simulink model "RobotX_ss_acoustics_1019_bbox"  (R2014a)
settings: Solver=FixedStepDiscrete  StartTime=0.0  StopTime=inf  FixedStep=.25  RelTol=1e-3
undefined symbols (not defined in the file): Com1, Com2, Com3, Com4, DiscIntNeverNeededParam, standard
libraries: xpcseriallib x14, dspmtrx3 x3, slrtlib x3, simulink x2, speedgoatlib x1, speedgoatlib_IO102 x1
(part 1 of 3)
settings Model: BufferReuse=off  Creator=wildcat  LastModifiedBy=wildcat
settings SolverCC: EnableConcurrentExecution=on
settings DataIOCC: SignalLoggingSaveFormat=ModelDataLogs
settings OptimizationCC: BlockReduction=off  OptimizeBlockIOStorage=off  BufferReuse=off  GlobalBufferReuse=off  ExpressionFolding=off  LocalBlockOutputs=off
settings DebuggingCC: UnderspecifiedInitializationDetection=Classic  StateNameClashWarn=warning
settings HardwareCC: ProdIntDivRoundTo=Zero  ProdEndianess=LittleEndian  ProdHWDeviceType=Generic->32-bit x86 compatible
settings RTWCC: SystemTargetFile=slrt.tlc  TemplateMakefile=slrt_default_tmf  Description=Simulink Real-Time  ProcessScript=slrt_make_rtw_hook  RTWCompilerOptimization=On
settings SimulinkRealTimeCC: GeneratePreprocessorConditionals=Disable all  EnableShiftOperators=on

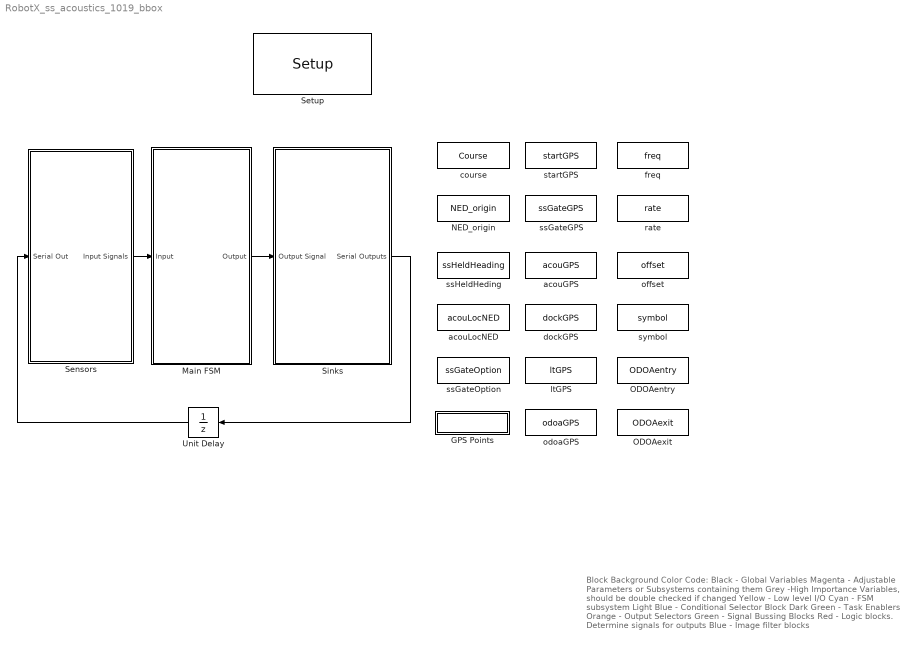
== system RobotX_ss_acoustics_1019_bbox ==
  note: Block Background Color Code:
      | Black - Global Variables
      | Magenta - Adjustable Parameters or Subsystems containing them
      | Grey -High Importance Variables, should be double checked if changed
      | Yellow - Low level I/O
      | Cyan - FSM subsystem
      | Light Blue - Conditional Selector Block
      | Dark Green - Task Enablers
      | Orange - Output Selectors
      | Green - Signal Bussing Blocks
      | Red - Logic blocks. Determine signals for outputs
      | Blue - Image filter blocks
  GPS Points : Subsystem
  Main FSM : Subsystem
  NED_origin : DataStoreMemory  DataStoreName=NED_origin  ReadBeforeWriteMsg=warning  WriteAfterWriteMsg=warning  WriteAfterReadMsg=warning  InitialValue="[1.2879,  103.8584]"  VectorParams1D=off
  ODOAentry : DataStoreMemory  DataStoreName=ODOAentry  ReadBeforeWriteMsg=warning  WriteAfterWriteMsg=warning  WriteAfterReadMsg=warning  VectorParams1D=off
  ODOAexit : DataStoreMemory  DataStoreName=ODOAexit  ReadBeforeWriteMsg=warning  WriteAfterWriteMsg=warning  WriteAfterReadMsg=warning  VectorParams1D=off
  Sensors : Subsystem
  Setup : speedgoatlib_IO102/Setup  group=Digital output setup  id=1  range=+-5V  cal=off  pciSlot=-1  adChannelMode=Multiple-channel (enter number of channels below)  adChannel=16  adCoupling=Differential  daChannel=[1,2,3,4]  daReset=[1]  daInitValue=[0]  diChannel=[1,2,3,4,5,6,7,8]  doChannel=[1,2,3,4,5,6,7,8]  doReset=[1]  doInitValue=[0]
  Sinks : Subsystem
  Unit Delay : UnitDelay  SampleTime=-1
  acouGPS : DataStoreMemory  DataStoreName=acouGPS  ReadBeforeWriteMsg=warning  WriteAfterWriteMsg=warning  WriteAfterReadMsg=warning  InitialValue=zeros(4,2)  VectorParams1D=off
  acouLocNED : DataStoreMemory  DataStoreName=acouLocNED  ReadBeforeWriteMsg=warning  WriteAfterWriteMsg=warning  WriteAfterReadMsg=warning  InitialValue=[45, -180; 60, -160; 75, -175]  VectorParams1D=off
  course : DataStoreMemory  DataStoreName=Course  ReadBeforeWriteMsg=warning  WriteAfterWriteMsg=warning  WriteAfterReadMsg=warning  InitialValue=uint8('A')  VectorParams1D=off
  dockGPS : DataStoreMemory  DataStoreName=dockGPS  ReadBeforeWriteMsg=warning  WriteAfterWriteMsg=warning  WriteAfterReadMsg=warning  InitialValue=zeros(4,2)  VectorParams1D=off
  freq : DataStoreMemory  DataStoreName=freq  ReadBeforeWriteMsg=warning  WriteAfterWriteMsg=warning  WriteAfterReadMsg=warning  VectorParams1D=off
  ltGPS : DataStoreMemory  DataStoreName=ltGPS  ReadBeforeWriteMsg=warning  WriteAfterWriteMsg=warning  WriteAfterReadMsg=warning  InitialValue=zeros(4,2)  VectorParams1D=off
  odoaGPS : DataStoreMemory  DataStoreName=odoaGPS  ReadBeforeWriteMsg=warning  WriteAfterWriteMsg=warning  WriteAfterReadMsg=warning  InitialValue=zeros(4,2)  VectorParams1D=off
  offset : DataStoreMemory  DataStoreName=offset  ReadBeforeWriteMsg=warning  WriteAfterWriteMsg=warning  WriteAfterReadMsg=warning  VectorParams1D=off
  rate : DataStoreMemory  DataStoreName=rate  ReadBeforeWriteMsg=warning  WriteAfterWriteMsg=warning  WriteAfterReadMsg=warning  VectorParams1D=off
  ssGateGPS : DataStoreMemory  DataStoreName=ssGateGPS  ReadBeforeWriteMsg=warning  WriteAfterWriteMsg=warning  WriteAfterReadMsg=warning  InitialValue=zeros(4,2)  VectorParams1D=off
  ssGateOption : DataStoreMemory  DataStoreName=ssGateOption  ReadBeforeWriteMsg=warning  WriteAfterWriteMsg=warning  WriteAfterReadMsg=warning  VectorParams1D=off
  ssHeldHeding : DataStoreMemory  DataStoreName=ssHeldHeading  ReadBeforeWriteMsg=warning  WriteAfterWriteMsg=warning  WriteAfterReadMsg=warning
  startGPS : DataStoreMemory  DataStoreName=startGPS  ReadBeforeWriteMsg=warning  WriteAfterWriteMsg=warning  WriteAfterReadMsg=warning  InitialValue=zeros(1,2)  VectorParams1D=off
  symbol : DataStoreMemory  DataStoreName=symbol  ReadBeforeWriteMsg=warning  WriteAfterWriteMsg=warning  WriteAfterReadMsg=warning  VectorParams1D=off
  wires:
  Main FSM/1(Output) -> Sinks/1(Output Signal)
  Sensors/1(Input Signals) -> Main FSM/1(Input)
  Sinks/1(Serial Outputs) -> Unit Delay/1
  Unit Delay/1 -> Sensors/1(Serial Out)

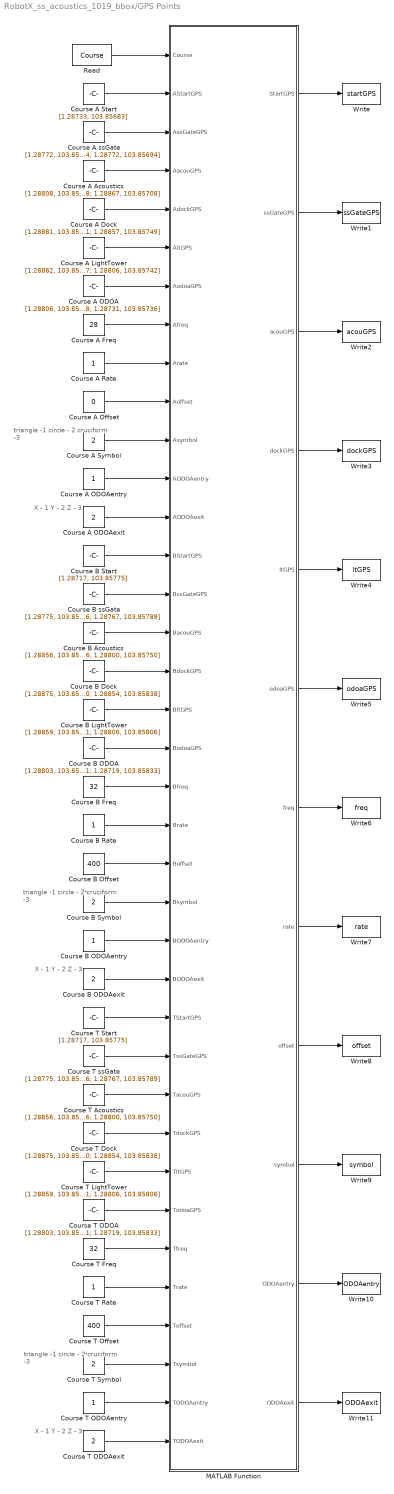
== system RobotX_ss_acoustics_1019_bbox/GPS Points ==
  note: X - 1
      | Y - 2
      | Z - 3
  note: triangle -1
      | circle - 2
      | cruciform -3
  note: X - 1
      | Y - 2
      | Z - 3
  note: triangle -1
      | circle - 2
      | cruciform -3
  note: X - 1
      | Y - 2
      | Z - 3
  note: triangle -1
      | circle - 2
      | cruciform -3
  Course A Acoustics : Constant  Value=[1.28808, 103.85714; 1.28869, 103.85669; 1.28817, 103.85658; 1.28867, 103.85708]  VectorParams1D=off
  Course A Dock : Constant  Value=[1.28881, 103.85717; 1.28875, 103.85753; 1.28862, 103.85721; 1.28857, 103.85749]  VectorParams1D=off
  Course A Freq : Constant  Value=28  VectorParams1D=off
  Course A LightTower : Constant  Value=[1.28862, 103.85721; 1.28857, 103.85749; 1.28806, 103.85717; 1.28806, 103.85742]  VectorParams1D=off
  Course A ODOA : Constant  Value=[1.28806, 103.85717; 1.28806, 103.85742; 1.28733, 103.85708; 1.28731, 103.85736]  VectorParams1D=off
  Course A ODOAentry : Constant  VectorParams1D=off
  Course A ODOAexit : Constant  Value=2  VectorParams1D=off
  Course A Offset : Constant  Value=0  VectorParams1D=off
  Course A Rate : Constant  VectorParams1D=off
  Course A Start : Constant  Value=[1.28733, 103.85683]  VectorParams1D=off
  Course A Symbol : Constant  Value=2  VectorParams1D=off
  Course A ssGate : Constant  Value=[1.28772, 103.85675; 1.28739, 103.85675; 1.28739, 103.85694; 1.28772, 103.85694]  VectorParams1D=off
  Course B Acoustics : Constant  Value=[1.28856, 103.85761; 1.28867, 103.85794; 1.28800, 103.85786; 1.28800, 103.85750]  VectorParams1D=off
  Course B Dock : Constant  Value=[1.28875, 103.85811; 1.28869, 103.85844; 1.28859, 103.85810; 1.28854, 103.85838]  VectorParams1D=off
  Course B Freq : Constant  Value=32  VectorParams1D=off
  Course B LightTower : Constant  Value=[1.28859, 103.85810; 1.28854, 103.85838; 1.28803, 103.85831; 1.28806, 103.85806]  VectorParams1D=off
  Course B ODOA : Constant  Value=[1.28803, 103.85831; 1.28806, 103.85806; 1.28722, 103.85811; 1.28719, 103.85833]  VectorParams1D=off
  Course B ODOAentry : Constant  VectorParams1D=off
  Course B ODOAexit : Constant  Value=2  VectorParams1D=off
  Course B Offset : Constant  Value=400  VectorParams1D=off
  Course B Rate : Constant  VectorParams1D=off
  Course B Start : Constant  Value=[1.28717, 103.85775]  VectorParams1D=off
  Course B Symbol : Constant  Value=2  VectorParams1D=off
  Course B ssGate : Constant  Value=[1.28775, 103.85761; 1.28725, 103.85764; 1.28719, 103.85786; 1.28767, 103.85789]  VectorParams1D=off
  Course T Acoustics : Constant  Value=[1.28856, 103.85761; 1.28867, 103.85794; 1.28800, 103.85786; 1.28800, 103.85750]  VectorParams1D=off
  Course T Dock : Constant  Value=[1.28875, 103.85811; 1.28869, 103.85844; 1.28859, 103.85810; 1.28854, 103.85838]  VectorParams1D=off
  Course T Freq : Constant  Value=32  VectorParams1D=off
  Course T LightTower : Constant  Value=[1.28859, 103.85810; 1.28854, 103.85838; 1.28803, 103.85831; 1.28806, 103.85806]  VectorParams1D=off
  Course T ODOA : Constant  Value=[1.28803, 103.85831; 1.28806, 103.85806; 1.28722, 103.85811; 1.28719, 103.85833]  VectorParams1D=off
  Course T ODOAentry : Constant  VectorParams1D=off
  Course T ODOAexit : Constant  Value=2  VectorParams1D=off
  Course T Offset : Constant  Value=400  VectorParams1D=off
  Course T Rate : Constant  VectorParams1D=off
  Course T Start : Constant  Value=[1.28717, 103.85775]  VectorParams1D=off
  Course T Symbol : Constant  Value=2  VectorParams1D=off
  Course T ssGate : Constant  Value=[1.28775, 103.85761; 1.28725, 103.85764; 1.28719, 103.85786; 1.28767, 103.85789]  VectorParams1D=off
  MATLAB Function : MATLAB Function  TreatAsAtomicUnit=on
  Read : DataStoreRead  DataStoreName=Course
  Write : DataStoreWrite  DataStoreName=startGPS
  Write1 : DataStoreWrite  DataStoreName=ssGateGPS
  Write10 : DataStoreWrite  DataStoreName=ODOAentry
  Write11 : DataStoreWrite  DataStoreName=ODOAexit
  Write2 : DataStoreWrite  DataStoreName=acouGPS
  Write3 : DataStoreWrite  DataStoreName=dockGPS
  Write4 : DataStoreWrite  DataStoreName=ltGPS
  Write5 : DataStoreWrite  DataStoreName=odoaGPS
  Write6 : DataStoreWrite  DataStoreName=freq
  Write7 : DataStoreWrite  DataStoreName=rate
  Write8 : DataStoreWrite  DataStoreName=offset
  Write9 : DataStoreWrite  DataStoreName=symbol
  wires:
  Course T LightTower/1 -> MATLAB Function/30(TltGPS)
  Course T Rate/1 -> MATLAB Function/33(Trate)
  Course T Symbol/1 -> MATLAB Function/35(Tsymbol)
  Course T ODOA/1 -> MATLAB Function/31(TodoaGPS)
  Course T Freq/1 -> MATLAB Function/32(Tfreq)
  Course T Offset/1 -> MATLAB Function/34(Toffset)
  Course T ODOAexit/1 -> MATLAB Function/37(TODOAexit)
  Course T Dock/1 -> MATLAB Function/29(TdockGPS)
  Course T Acoustics/1 -> MATLAB Function/28(TacouGPS)
  Course T ODOAentry/1 -> MATLAB Function/36(TODOAentry)
  Course T Start/1 -> MATLAB Function/26(TStartGPS)
  Course T ssGate/1 -> MATLAB Function/27(TssGateGPS)
  Course B ODOAexit/1 -> MATLAB Function/25(BODOAexit)
  Course B Dock/1 -> MATLAB Function/17(BdockGPS)
  Course B Rate/1 -> MATLAB Function/21(Brate)
  Course B LightTower/1 -> MATLAB Function/18(BltGPS)
  Course B Freq/1 -> MATLAB Function/20(Bfreq)
  Course B Symbol/1 -> MATLAB Function/23(Bsymbol)
  Course B ODOA/1 -> MATLAB Function/19(BodoaGPS)
  Course B ODOAentry/1 -> MATLAB Function/24(BODOAentry)
  Course B Acoustics/1 -> MATLAB Function/16(BacouGPS)
  Course B Offset/1 -> MATLAB Function/22(Boffset)
  Course B Start/1 -> MATLAB Function/14(BStartGPS)
  Course B ssGate/1 -> MATLAB Function/15(BssGateGPS)
  Course A ODOAentry/1 -> MATLAB Function/12(AODOAentry)
  Course A Acoustics/1 -> MATLAB Function/4(AacouGPS)
  Course A Offset/1 -> MATLAB Function/10(Aoffset)
  Course A Dock/1 -> MATLAB Function/5(AdockGPS)
  Course A Freq/1 -> MATLAB Function/8(Afreq)
  Course A Rate/1 -> MATLAB Function/9(Arate)
  Course A LightTower/1 -> MATLAB Function/6(AltGPS)
  Course A ODOAexit/1 -> MATLAB Function/13(AODOAexit)
  Course A ODOA/1 -> MATLAB Function/7(AodoaGPS)
  Course A Symbol/1 -> MATLAB Function/11(Asymbol)
  Course A ssGate/1 -> MATLAB Function/3(AssGateGPS)
  Course A Start/1 -> MATLAB Function/2(AStartGPS)
  Read/1 -> MATLAB Function/1(Course)
  MATLAB Function/1(StartGPS) -> Write/1
  MATLAB Function/2(ssGateGPS) -> Write1/1
  MATLAB Function/3(acouGPS) -> Write2/1
  MATLAB Function/4(dockGPS) -> Write3/1
  MATLAB Function/5(ltGPS) -> Write4/1
  MATLAB Function/6(odoaGPS) -> Write5/1
  MATLAB Function/7(freq) -> Write6/1
  MATLAB Function/8(rate) -> Write7/1
  MATLAB Function/9(offset) -> Write8/1
  MATLAB Function/10(symbol) -> Write9/1
  MATLAB Function/11(ODOAentry) -> Write10/1
  MATLAB Function/12(ODOAexit) -> Write11/1

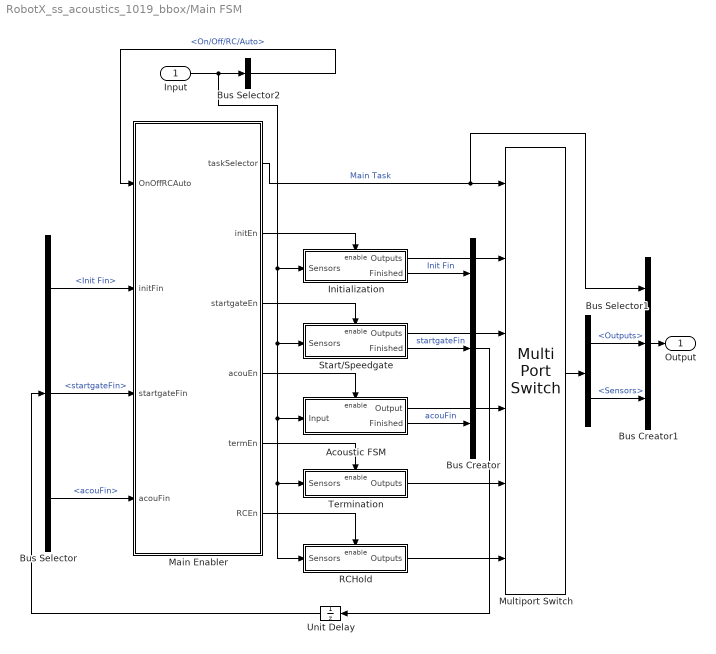
== system RobotX_ss_acoustics_1019_bbox/Main FSM ==
  Input : Inport
  Acoustic FSM : Subsystem
  Bus Creator : BusCreator  Inputs=3
  Bus Creator1 : BusCreator  Inputs=3
  Bus Selector : BusSelector  OutputSignals=Init Fin,startgateFin,acouFin
  Bus Selector1 : BusSelector  OutputSignals=Outputs,Sensors
  Bus Selector2 : BusSelector  OutputSignals=Navigation Message.On/Off/RC/Auto
  Initialization : Subsystem
  Main Enabler : MATLAB Function  TreatAsAtomicUnit=on
  Multiport Switch : MultiPortSwitch  Inputs=5
  RCHold : Subsystem
  Start/Speedgate : Subsystem  TreatAsAtomicUnit=on
  Termination : Subsystem
  Unit Delay : UnitDelay  SampleTime=-1
  Output : Outport
  wires:
  Input/1 -> Initialization/1(Sensors), Acoustic FSM/1(Input), Termination/1(Sensors), RCHold/1(Sensors), Start/Speedgate/1(Sensors), Bus Selector2/1
  Bus Selector2/1 -> Main Enabler/1(OnOffRCAuto)  "<On/Off/RC/Auto>"
  RCHold/1(Outputs) -> Multiport Switch/6
  Main Enabler/2(initEn) -> Initialization/Enable
  Main Enabler/3(startgateEn) -> Start/Speedgate/Enable
  Main Enabler/6(RCEn) -> RCHold/Enable
  Main Enabler/1(taskSelector) -> Bus Creator1/1, Multiport Switch/1  "Main Task"
  Multiport Switch/1 -> Bus Selector1/1
  Unit Delay/1 -> Bus Selector/1
  Termination/1(Outputs) -> Multiport Switch/5
  Main Enabler/5(termEn) -> Termination/Enable
  Bus Creator/1 -> Unit Delay/1
  Bus Selector/1 -> Main Enabler/2(initFin)  "<Init Fin>"
  Bus Selector/2 -> Main Enabler/3(startgateFin)  "<startgateFin>"
  Acoustic FSM/1(Output) -> Multiport Switch/4
  Main Enabler/4(acouEn) -> Acoustic FSM/Enable
  Start/Speedgate/1(Outputs) -> Multiport Switch/3
  Initialization/1(Outputs) -> Multiport Switch/2
  Initialization/2(Finished) -> Bus Creator/1  "Init Fin"
  Start/Speedgate/2(Finished) -> Bus Creator/2  "startgateFin"
  Acoustic FSM/2(Finished) -> Bus Creator/3  "acouFin"
  Bus Selector/3 -> Main Enabler/4(acouFin)  "<acouFin>"
  Bus Creator1/1 -> Output/1
  Bus Selector1/1 -> Bus Creator1/2  "<Outputs>"
  Bus Selector1/2 -> Bus Creator1/3  "<Sensors>"

== system RobotX_ss_acoustics_1019_bbox/Sensors ==
  Serial Out : Inport
  Serial In : Subsystem
  Input Signals : Outport
  wires:
  Serial In/1(Serial In) -> Input Signals/1  "Sensors"
  Serial Out/1 -> Serial In/1(Serial Out)

== system RobotX_ss_acoustics_1019_bbox/Sinks ==
  Output Signal : Inport
  Serial Outputs : Outport
  wires:
  Output Signal/1 -> Serial Outputs/1

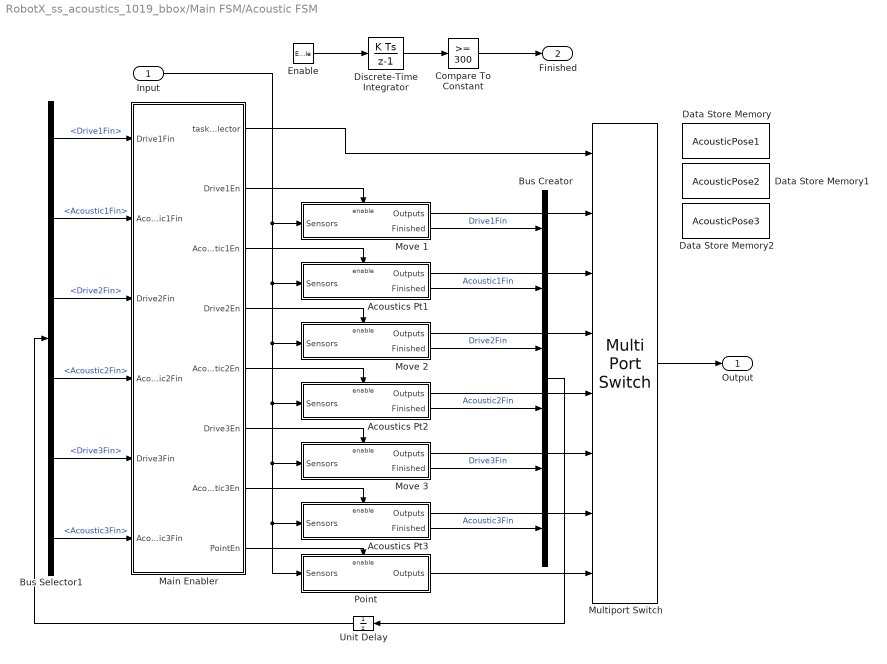
== system RobotX_ss_acoustics_1019_bbox/Main FSM/Acoustic FSM ==
  Input : Inport
  Enable : EnablePort  ShowOutputPort=on
  Acoustics Pt1 : Subsystem  TreatAsAtomicUnit=on
  Acoustics Pt2 : Subsystem  TreatAsAtomicUnit=on
  Acoustics Pt3 : Subsystem  TreatAsAtomicUnit=on
  Bus Creator : BusCreator  Inputs=6
  Bus Selector1 : BusSelector  OutputSignals=Drive1Fin,Acoustic1Fin,Drive2Fin,Acoustic2Fin,Drive3Fin,Acoustic3Fin
  Compare To Constant : simulink/Logic and Bit Operations/Compare To Constant  relop=>=  const=300  OutDataTypeStr=boolean
  Data Store Memory : DataStoreMemory  DataStoreName=AcousticPose1  ReadBeforeWriteMsg=warning  WriteAfterWriteMsg=warning  WriteAfterReadMsg=warning  InitialValue=[0 0 0]
  Data Store Memory1 : DataStoreMemory  DataStoreName=AcousticPose2  ReadBeforeWriteMsg=warning  WriteAfterWriteMsg=warning  WriteAfterReadMsg=warning  InitialValue=[0 0 0]
  Data Store Memory2 : DataStoreMemory  DataStoreName=AcousticPose3  ReadBeforeWriteMsg=warning  WriteAfterWriteMsg=warning  WriteAfterReadMsg=warning  InitialValue=[0 0 0]
  Discrete-Time Integrator : DiscreteIntegrator  SampleTime=-1  ICPrevOutput=DiscIntNeverNeededParam  ICPrevScaledInput=DiscIntNeverNeededParam
  Main Enabler : MATLAB Function  TreatAsAtomicUnit=on
  Move 1 : Subsystem
  Move 2 : Subsystem
  Move 3 : Subsystem
  Multiport Switch : MultiPortSwitch  Inputs=7
  Point : Subsystem  TreatAsAtomicUnit=on
  Unit Delay : UnitDelay  SampleTime=-1
  Output : Outport
  Finished : Outport  Port=2
  wires:
  Input/1 -> Move 1/1(Sensors), Acoustics Pt1/1(Sensors), Move 2/1(Sensors), Acoustics Pt2/1(Sensors), Move 3/1(Sensors), Acoustics Pt3/1(Sensors), Point/1(Sensors)
  Multiport Switch/1 -> Output/1
  Unit Delay/1 -> Bus Selector1/1
  Move 1/1(Outputs) -> Multiport Switch/2
  Move 1/2(Finished) -> Bus Creator/1  "Drive1Fin"
  Acoustics Pt1/2(Finished) -> Bus Creator/2  "Acoustic1Fin"
  Move 2/2(Finished) -> Bus Creator/3  "Drive2Fin"
  Acoustics Pt2/2(Finished) -> Bus Creator/4  "Acoustic2Fin"
  Move 3/2(Finished) -> Bus Creator/5  "Drive3Fin"
  Acoustics Pt3/2(Finished) -> Bus Creator/6  "Acoustic3Fin"
  Bus Creator/1 -> Unit Delay/1
  Main Enabler/2(Drive1En) -> Move 1/Enable
  Main Enabler/3(Acoustic1En) -> Acoustics Pt1/Enable
  Main Enabler/4(Drive2En) -> Move 2/Enable
  Main Enabler/5(Acoustic2En) -> Acoustics Pt2/Enable
  Main Enabler/6(Drive3En) -> Move 3/Enable
  Main Enabler/7(Acoustic3En) -> Acoustics Pt3/Enable
  Main Enabler/8(PointEn) -> Point/Enable
  Bus Selector1/6 -> Main Enabler/6(Acoustic3Fin)  "<Acoustic3Fin>"
  Bus Selector1/4 -> Main Enabler/4(Acoustic2Fin)  "<Acoustic2Fin>"
  Bus Selector1/2 -> Main Enabler/2(Acoustic1Fin)  "<Acoustic1Fin>"
  Bus Selector1/5 -> Main Enabler/5(Drive3Fin)  "<Drive3Fin>"
  Bus Selector1/3 -> Main Enabler/3(Drive2Fin)  "<Drive2Fin>"
  Bus Selector1/1 -> Main Enabler/1(Drive1Fin)  "<Drive1Fin>"
  Acoustics Pt1/1(Outputs) -> Multiport Switch/3
  Move 2/1(Outputs) -> Multiport Switch/4
  Acoustics Pt2/1(Outputs) -> Multiport Switch/5
  Move 3/1(Outputs) -> Multiport Switch/6
  Acoustics Pt3/1(Outputs) -> Multiport Switch/7
  Point/1(Outputs) -> Multiport Switch/8
  Main Enabler/1(taskSelector) -> Multiport Switch/1
  Enable/1 -> Discrete-Time Integrator/1
  Discrete-Time Integrator/1 -> Compare To Constant/1
  Compare To Constant/1 -> Finished/1

== system RobotX_ss_acoustics_1019_bbox/Main FSM/Initialization ==
  Sensors : Inport
  Enable : EnablePort  ShowOutputPort=on
  Compare To Constant : simulink/Logic and Bit Operations/Compare To Constant  relop=>=  const=50  OutDataTypeStr=boolean
  Data Type Conversion : DataTypeConversion  OutDataTypeStr=double
  Discrete-Time Integrator : DiscreteIntegrator  SampleTime=-1  ICPrevOutput=DiscIntNeverNeededParam  ICPrevScaledInput=DiscIntNeverNeededParam
  Output Heirarchy : Subsystem
  Outputs : Outport
  Finished : Outport  Port=2
  wires:
  Sensors/1 -> Output Heirarchy/1(Sensors)
  Output Heirarchy/1(Outputs) -> Outputs/1
  Compare To Constant/1 -> Data Type Conversion/1
  Enable/1 -> Discrete-Time Integrator/1
  Discrete-Time Integrator/1 -> Compare To Constant/1
  Data Type Conversion/1 -> Finished/1

== system RobotX_ss_acoustics_1019_bbox/Main FSM/RCHold ==
  Sensors : Inport
  Enable : EnablePort
  Direct Control : Subsystem
  Outputs : Outport
  wires:
  Direct Control/1(Outputs) -> Outputs/1
  Sensors/1 -> Direct Control/1(Sensors)

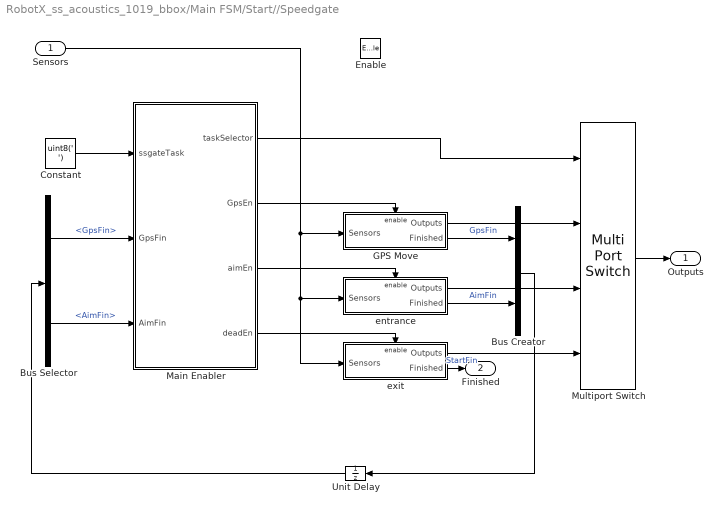
== system RobotX_ss_acoustics_1019_bbox/Main FSM/Start//Speedgate ==
  Sensors : Inport
  Enable : EnablePort
  Bus Creator : BusCreator  Inputs=2
  Bus Selector : BusSelector  OutputSignals=GpsFin,AimFin
  Constant : Constant  Value=uint8(' ')  VectorParams1D=off
  GPS Move : Subsystem
  Main Enabler : MATLAB Function  TreatAsAtomicUnit=on
  Multiport Switch : MultiPortSwitch
  Unit Delay : UnitDelay  SampleTime=-1
  entrance : Subsystem
  exit : Subsystem
  Outputs : Outport
  Finished : Outport  Port=2  InitialOutput=0
  wires:
  Main Enabler/1(taskSelector) -> Multiport Switch/1
  Constant/1 -> Main Enabler/1(ssgateTask)
  Bus Selector/1 -> Main Enabler/2(GpsFin)  "<GpsFin>"
  Unit Delay/1 -> Bus Selector/1
  Main Enabler/2(GpsEn) -> GPS Move/Enable
  Main Enabler/4(deadEn) -> exit/Enable
  Bus Creator/1 -> Unit Delay/1
  Sensors/1 -> exit/1(Sensors), entrance/1(Sensors), GPS Move/1(Sensors)
  Multiport Switch/1 -> Outputs/1
  Main Enabler/3(aimEn) -> entrance/Enable
  exit/1(Outputs) -> Multiport Switch/4
  entrance/1(Outputs) -> Multiport Switch/3
  GPS Move/1(Outputs) -> Multiport Switch/2
  GPS Move/2(Finished) -> Bus Creator/1  "GpsFin"
  entrance/2(Finished) -> Bus Creator/2  "AimFin"
  Bus Selector/2 -> Main Enabler/3(AimFin)  "<AimFin>"
  exit/2(Finished) -> Finished/1  "StartFin"

== system RobotX_ss_acoustics_1019_bbox/Main FSM/Termination ==
  Sensors : Inport
  Enable : EnablePort
  Bus Selector : BusSelector  OutputSignals=Navigation Message.Pose.X,Navigation Message.Pose.Y,Navigation Message.Pose.Psi,Navigation Message.Velocity.u
  CalcTimes : MATLAB Function  TreatAsAtomicUnit=on
  Data Store Read : DataStoreRead  DataStoreName=startGPS
  Data Store Read1 : DataStoreRead  DataStoreName=NED_origin
  GPSMove : MATLAB Function  TreatAsAtomicUnit=on
  LLA to NED : MATLAB Function  TreatAsAtomicUnit=on
  Output Reassign : Subsystem
  Outputs : Outport
  wires:
  GPSMove/2(pts) -> CalcTimes/1(pts)
  Sensors/1 -> Output Reassign/3(Sensors), Bus Selector/1
  Bus Selector/1 -> GPSMove/2(X)  "<X>"
  Bus Selector/2 -> GPSMove/3(Y)  "<Y>"
  Bus Selector/3 -> GPSMove/4(Psi)  "<Psi>"
  Bus Selector/4 -> CalcTimes/2(u)  "<u>"
  Output Reassign/1(Outputs) -> Outputs/1
  CalcTimes/1(Data) -> Output Reassign/2(Data)
  GPSMove/1(valid) -> Output Reassign/1(Vaild)
  LLA to NED/1(GoalNED) -> GPSMove/1(GoalNED)
  Data Store Read/1 -> LLA to NED/1(GoalLLA)
  Data Store Read1/1 -> LLA to NED/2(NED_origin)

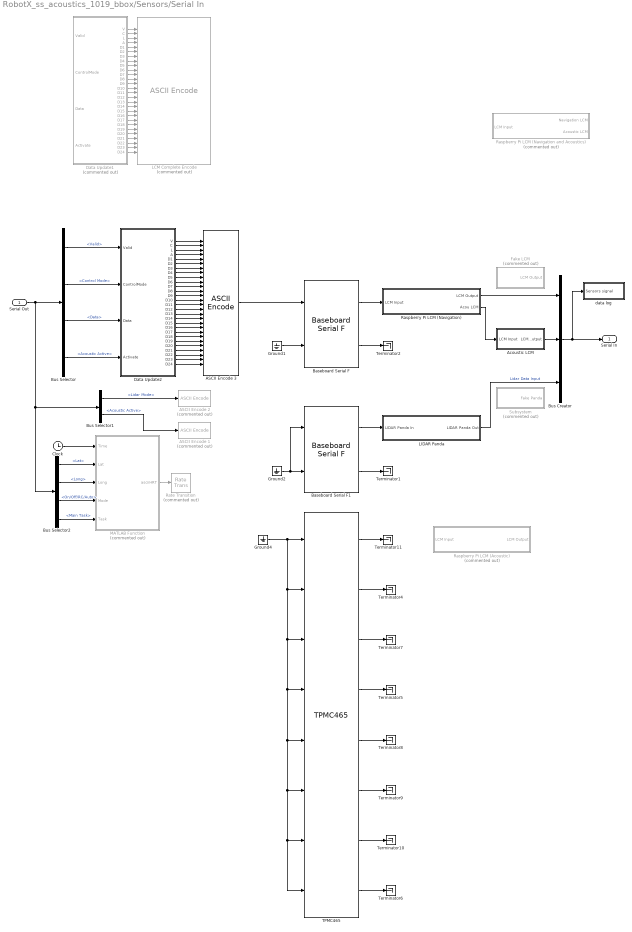
== system RobotX_ss_acoustics_1019_bbox/Sensors/Serial In ==
  Serial Out : Inport
  " Raspberry Pi LCM (Acoustic)" : Subsystem  Commented=on
  " Raspberry Pi LCM (Navigation and Acoustics)" : Subsystem  Commented=on
  " Raspberry Pi LCM (Navigation)" : Subsystem
  ASCII Encode 1 : xpcseriallib/ASCII Encode   Commented=on  format="{\"Activate\":%d} \\r\\n"  nvars=1  maxlength=20  vartypes={ 'double' }
  ASCII Encode 2 : xpcseriallib/ASCII Encode   Commented=on  format=SGTask:%d \r\n  nvars=1  maxlength=128  vartypes={ 'double' }
  ASCII Encode 3 : xpcseriallib/ASCII Encode   format="{\"Valid\":%d, \"Mode\":%d, \"Length\":%d, \"Activate\":%d, \"Waypoints\":[%f, %f, %f, %f, %f, %f, %f, %f, %f, %f, %f, %f, %f, %f, %f, %f, %f, %f, %f, %f, %f, %f, %f, %f]} \\r\\n"  nvars=28  maxlength=1000  vartypes={ 'double' }
  Acoustic LCM : Subsystem
  Baseboard Serial F : xpcseriallib/Mainboard/Baseboard Serial F  group=Basic Setup  port=1  irqnum=4  saddr1=0x3f8  saddr2=0x3e8  config=Com1/Com3  baud1=115200  parity1=Even  ndata1=7  nstop1=1  fifomode1=64 deep  rlevel1=quarter full  automode1=on  xmtfifosize1=1024  xmtdatatype1=8 bit uint null terminated  rcvfifosize1=1024  baud2=115200  parity2=Even  ndata2=7  nstop2=1  fifomode2=64 deep  rlevel2=1  automode2=on  xmtfifosize2=1024  xmtdatatype2=8 bit uint null terminated  rcvfifosize2=1024
  Baseboard Serial F1 : xpcseriallib/Mainboard/Baseboard Serial F  group=Basic Setup  port=2  irqnum=4  saddr1=0x3f8  saddr2=0x3e8  config=Com2/Com4  baud1=115200  parity1=Even  ndata1=7  nstop1=1  fifomode1=64 deep  rlevel1=quarter full  automode1=on  xmtfifosize1=1024  xmtdatatype1=8 bit uint null terminated  rcvfifosize1=1024  baud2=115200  parity2=Even  ndata2=7  nstop2=1  fifomode2=64 deep  rlevel2=quarter full  automode2=on  xmtfifosize2=1024  xmtdatatype2=8 bit uint null terminated  rcvfifosize2=1024
  Bus Creator : BusCreator  Inputs=3
  Bus Selector : BusSelector  OutputSignals=Outputs.Navigation Outputs.Valid,Outputs.Navigation Outputs.Control Mode,Outputs.Navigation Outputs.Data,Outputs.Acoustic Active
  Bus Selector1 : BusSelector  OutputSignals=Outputs.Lidar Mode,Outputs.Acoustic Active
  Bus Selector2 : BusSelector  OutputSignals=Sensors.Navigation Message.GPS (LLA).Lat,Sensors.Navigation Message.GPS (LLA).Long,Sensors.Navigation Message.On/Off/RC/Auto,Main Task
  Clock : Clock
  Data Update1 : MATLAB Function  Commented=on  TreatAsAtomicUnit=on
  Data Update2 : MATLAB Function  TreatAsAtomicUnit=on
  Fake LCM : Subsystem  Commented=on
  Ground1 : Ground
  Ground2 : Ground
  Ground4 : Ground
  LCM Complete Encode : xpcseriallib/ASCII Encode   Commented=on  format="{\"Valid\":%d, \"Mode\":%d, \"Length\":%d, \"Activate\":%d, \"Waypoints\":[%f, %f, %f, %f, %f, %f, %f, %f, %f, %f, %f, %f, %f, %f, %f, %f, %f, %f, %f, %f, %f, %f, %f, %f]} \\r\\n"  nvars=28  maxlength=1000  vartypes={ 'double' }
  LIDAR Panda : Subsystem
  MATLAB Function : MATLAB Function  Commented=on  TreatAsAtomicUnit=on
  Rate Transition : RateTransition  Commented=on  Deterministic=off  OutPortSampleTime=1
  Subsystem : Subsystem  Commented=on
  TPMC465 : speedgoatlib/IO504/TPMC465  group=Basic Setup  port=2  irqnum=9  slot=-1  transceiver1=RS232 (max 921.6kb/s)  standard1=on  baud1=115200  bauddivisor1=1  sampling1=16x (standard)  prescale1=off  parity1=Even  ndata1=7  nstop1=1  rlevel1=half full (32)  hwmode1=none  swmode1=none  xonchar1=17  xoffchar1=19  rs485auto1=off  rs485delay1=0  xmtfifosize1=1024  xmtdatatype1=8 bit uint null terminated  rcvfifosize1=1024  transceiver2=RS232 (max 921.6kb/s)  standard2=on  baud2=115200  bauddivisor2=1  sampling2=16x (standard)  prescale2=off  parity2=Even  ndata2=7  nstop2=1  rlevel2=1  hwmode2=none  swmode2=none  xonchar2=17  xoffchar2=19  rs485auto2=off  rs485delay2=0  xmtfifosize2=1024  xmtdatatype2=8 bit uint null terminated  rcvfifosize2=1024  transceiver3=RS232 (max 921.6kb/s)  standard3=on  baud3=115200  bauddivisor3=1  sampling3=16x (standard)  prescale3=off  parity3=None  ndata3=8  nstop3=1  rlevel3=half full (32)  hwmode3=none  swmode3=none  xonchar3=17  xoffchar3=19  rs485auto3=off  rs485delay3=0  xmtfifosize3=1024  xmtdatatype3=8 bit uint null terminated  rcvfifosize3=1024  transceiver4=RS232 (max 921.6kb/s)  standard4=on  baud4=115200  bauddivisor4=1  sampling4=16x (standard)  prescale4=off  parity4=None  ndata4=8  nstop4=1  rlevel4=half full (32)  hwmode4=none  swmode4=none  xonchar4=17  xoffchar4=19  rs485auto4=off  rs485delay4=0  xmtfifosize4=1024  xmtdatatype4=8 bit uint null terminated  rcvfifosize4=1024  transceiver5=RS232 (max 921.6kb/s)  standard5=on  baud5=115200  bauddivisor5=1  sampling5=16x (standard)  prescale5=off  parity5=None  ndata5=8  nstop5=1  rlevel5=1  hwmode5=none  swmode5=none  xonchar5=17  xoffchar5=19  rs485auto5=off  rs485delay5=0  xmtfifosize5=1024  xmtdatatype5=8 bit uint null terminated  rcvfifosize5=1024  transceiver6=RS232 (max 921.6kb/s)  standard6=on  baud6=115200  bauddivisor6=1  sampling6=16x (standard)  prescale6=off  parity6=None  ndata6=8  nstop6=1  rlevel6=1  hwmode6=none  swmode6=none  xonchar6=17  xoffchar6=19  rs485auto6=off  rs485delay6=0  xmtfifosize6=1024  xmtdatatype6=8 bit uint null terminated  rcvfifosize6=1024  transceiver7=RS232 (max 921.6kb/s)  standard7=on  baud7=115200  bauddivisor7=1  sampling7=16x (standard)  prescale7=off  parity7=None  ndata7=8  nstop7=1  rlevel7=1  hwmode7=none  swmode7=none  xonchar7=17  xoffchar7=19  rs485auto7=off  rs485delay7=0  xmtfifosize7=1024  xmtdatatype7=8 bit uint null terminated  rcvfifosize7=1024  transceiver8=RS232 (max 921.6kb/s)  standard8=on  baud8=115200  bauddivisor8=1  sampling8=16x (standard)  prescale8=off  parity8=None  ndata8=8  nstop8=1  rlevel8=1  hwmode8=none  swmode8=none  xonchar8=17  xoffchar8=19  rs485auto8=off  rs485delay8=0  xmtfifosize8=1024  xmtdatatype8=8 bit uint null terminated  rcvfifosize8=1024
  Terminator{1..2,4..11} (10 alike) : Terminator
  data log : Subsystem
  Serial In : Outport
  wires:
  Baseboard Serial F1/1 -> LIDAR Panda/1(LIDAR Panda In)
  Serial Out/1 -> Bus Selector2/1, Bus Selector1/1, Bus Selector/1
  Baseboard Serial F/1 -> " Raspberry Pi LCM (Navigation)"/1(LCM Input)
  TPMC465/1 -> Terminator11/1
  ASCII Encode 3/1 -> Baseboard Serial F/1
  " Raspberry Pi LCM (Navigation)"/1(LCM Output) -> Bus Creator/1
  Bus Selector/1 -> Data Update2/1(Valid)  "<Valid>"
  Bus Selector/2 -> Data Update2/2(ControlMode)  "<Control Mode>"
  Bus Selector/3 -> Data Update2/3(Data)  "<Data>"
  Acoustic LCM/1(LCM Output) -> Bus Creator/2
  Bus Selector1/2 -> ASCII Encode 1/1  "<Acoustic Active>"
  Baseboard Serial F/2 -> Terminator2/1
  Ground1/1 -> Baseboard Serial F/2
  Bus Selector1/1 -> ASCII Encode 2/1  "<Lidar Mode>"
  Ground2/1 -> Baseboard Serial F1/1, Baseboard Serial F1/2
  LIDAR Panda/1(LIDAR Panda Out) -> Bus Creator/3  "Lidar Data Input"
  TPMC465/7 -> Terminator10/1
  TPMC465/5 -> Terminator8/1
  TPMC465/6 -> Terminator9/1
  TPMC465/3 -> Terminator7/1
  TPMC465/4 -> Terminator5/1
  TPMC465/8 -> Terminator6/1
  Ground4/1 -> TPMC465/3, TPMC465/4, TPMC465/5, TPMC465/6, TPMC465/7, TPMC465/8, TPMC465/2, TPMC465/1
  Baseboard Serial F1/2 -> Terminator1/1
  Bus Creator/1 -> Serial In/1, data log/1(Sensors signal)
  MATLAB Function/1(asciiHRT) -> Rate Transition/1
  Bus Selector2/4 -> MATLAB Function/5(Task)  "<Main Task>"
  Bus Selector2/3 -> MATLAB Function/4(Mode)  "<On/Off/RC/Auto>"
  Bus Selector2/2 -> MATLAB Function/3(Long)  "<Long>"
  Bus Selector2/1 -> MATLAB Function/2(Lat)  "<Lat>"
  TPMC465/2 -> Terminator4/1
  Clock/1 -> MATLAB Function/1(Time)
  Data Update1/1(V) -> LCM Complete Encode/1
  Data Update1/2(C) -> LCM Complete Encode/2
  Data Update1/6(D2) -> LCM Complete Encode/6
  Data Update1/7(D3) -> LCM Complete Encode/7
  Data Update1/8(D4) -> LCM Complete Encode/8
  Data Update1/5(D1) -> LCM Complete Encode/5
  Data Update1/9(D5) -> LCM Complete Encode/9
  Data Update1/10(D6) -> LCM Complete Encode/10
  Data Update1/11(D7) -> LCM Complete Encode/11
  Data Update1/12(D8) -> LCM Complete Encode/12
  Data Update1/13(D9) -> LCM Complete Encode/13
  Data Update1/18(D14) -> LCM Complete Encode/18
  Data Update1/15(D11) -> LCM Complete Encode/15
  Data Update1/20(D16) -> LCM Complete Encode/20
  Data Update1/21(D17) -> LCM Complete Encode/21
  Data Update1/19(D15) -> LCM Complete Encode/19
  Data Update1/14(D10) -> LCM Complete Encode/14
  Data Update1/16(D12) -> LCM Complete Encode/16
  Data Update1/22(D18) -> LCM Complete Encode/22
  Data Update1/23(D19) -> LCM Complete Encode/23
  Data Update1/24(D20) -> LCM Complete Encode/24
  Data Update1/25(D21) -> LCM Complete Encode/25
  Data Update1/27(D23) -> LCM Complete Encode/27
  Data Update1/26(D22) -> LCM Complete Encode/26
  Data Update1/28(D24) -> LCM Complete Encode/28
  Data Update1/3(L) -> LCM Complete Encode/3
  Data Update1/4(A) -> LCM Complete Encode/4
  Data Update1/17(D13) -> LCM Complete Encode/17
  " Raspberry Pi LCM (Navigation)"/2(Acou LCM) -> Acoustic LCM/1(LCM Input)
  Data Update2/21(D17) -> ASCII Encode 3/21
  Data Update2/20(D16) -> ASCII Encode 3/20
  Data Update2/19(D15) -> ASCII Encode 3/19
  Data Update2/4(A) -> ASCII Encode 3/4
  Data Update2/2(C) -> ASCII Encode 3/2
  Data Update2/18(D14) -> ASCII Encode 3/18
  Data Update2/16(D12) -> ASCII Encode 3/16
  Data Update2/7(D3) -> ASCII Encode 3/7
  Data Update2/6(D2) -> ASCII Encode 3/6
  Data Update2/5(D1) -> ASCII Encode 3/5
  Data Update2/17(D13) -> ASCII Encode 3/17
  Data Update2/9(D5) -> ASCII Encode 3/9
  Data Update2/10(D6) -> ASCII Encode 3/10
  Data Update2/24(D20) -> ASCII Encode 3/24
  Data Update2/23(D19) -> ASCII Encode 3/23
  Data Update2/28(D24) -> ASCII Encode 3/28
  Data Update2/26(D22) -> ASCII Encode 3/26
  Data Update2/25(D21) -> ASCII Encode 3/25
  Data Update2/3(L) -> ASCII Encode 3/3
  Data Update2/27(D23) -> ASCII Encode 3/27
  Data Update2/8(D4) -> ASCII Encode 3/8
  Data Update2/11(D7) -> ASCII Encode 3/11
  Data Update2/13(D9) -> ASCII Encode 3/13
  Data Update2/12(D8) -> ASCII Encode 3/12
  Data Update2/14(D10) -> ASCII Encode 3/14
  Data Update2/22(D18) -> ASCII Encode 3/22
  Data Update2/15(D11) -> ASCII Encode 3/15
  Bus Selector/4 -> Data Update2/4(Activate)  "<Acoustic Active>"
  Data Update2/1(V) -> ASCII Encode 3/1

== system RobotX_ss_acoustics_1019_bbox/Main FSM/Acoustic FSM/Acoustics Pt1 ==
  Sensors : Inport
  Enable : EnablePort
  Bus Selector : BusSelector  OutputSignals=Acoustic Message.Deployed,Navigation Message.Pose.X,Navigation Message.Pose.Y,Navigation Message.Pose.Psi,Acoustic Message.Bearings.Horizontal Bearing,Acoustic Message.Elapsed Time
  Data Store Write : DataStoreWrite  DataStoreName=AcousticPose1
  Output Heirarchy : Subsystem
  Ping Point : MATLAB Function  TreatAsAtomicUnit=on
  Outputs : Outport
  Finished : Outport  Port=2
  wires:
  Sensors/1 -> Output Heirarchy/2(Sensors), Bus Selector/1
  Ping Point/3(Data) -> Output Heirarchy/1(Data)
  Output Heirarchy/1(Outputs) -> Outputs/1
  Bus Selector/3 -> Ping Point/3(Y)  "<Y>"
  Bus Selector/2 -> Ping Point/2(X)  "<X>"
  Bus Selector/4 -> Ping Point/4(Psi)  "<Psi>"
  Bus Selector/5 -> Ping Point/5(HorizBearing)  "<Horizontal Bearing>"
  Ping Point/2(Finished) -> Finished/1
  Ping Point/1(acousticPose) -> Data Store Write/1
  Bus Selector/1 -> Ping Point/1(Deployed)  "<Deployed>"
  Bus Selector/6 -> Ping Point/6(ElapsedTime)  "<Elapsed Time>"

== system RobotX_ss_acoustics_1019_bbox/Main FSM/Acoustic FSM/Acoustics Pt2 ==
  Sensors : Inport
  Enable : EnablePort
  Bus Selector : BusSelector  OutputSignals=Acoustic Message.Deployed,Navigation Message.Pose.X,Navigation Message.Pose.Y,Navigation Message.Pose.Psi,Acoustic Message.Bearings.Horizontal Bearing,Acoustic Message.Elapsed Time
  Data Store Write : DataStoreWrite  DataStoreName=AcousticPose2
  Output Heirarchy : Subsystem
  Ping Point : MATLAB Function  TreatAsAtomicUnit=on
  Outputs : Outport
  Finished : Outport  Port=2
  wires:
  Sensors/1 -> Output Heirarchy/2(Sensors), Bus Selector/1
  Ping Point/3(Data) -> Output Heirarchy/1(Data)
  Output Heirarchy/1(Outputs) -> Outputs/1
  Bus Selector/3 -> Ping Point/3(Y)  "<Y>"
  Bus Selector/2 -> Ping Point/2(X)  "<X>"
  Bus Selector/4 -> Ping Point/4(Psi)  "<Psi>"
  Bus Selector/5 -> Ping Point/5(HorizBearing)  "<Horizontal Bearing>"
  Ping Point/2(Finished) -> Finished/1
  Ping Point/1(acousticPose) -> Data Store Write/1
  Bus Selector/1 -> Ping Point/1(Deployed)  "<Deployed>"
  Bus Selector/6 -> Ping Point/6(ElapsedTime)  "<Elapsed Time>"

== system RobotX_ss_acoustics_1019_bbox/Main FSM/Acoustic FSM/Acoustics Pt3 ==
  Sensors : Inport
  Enable : EnablePort
  Bus Selector : BusSelector  OutputSignals=Acoustic Message.Deployed,Navigation Message.Pose.X,Navigation Message.Pose.Y,Navigation Message.Pose.Psi,Acoustic Message.Bearings.Horizontal Bearing,Acoustic Message.Elapsed Time
  Data Store Write : DataStoreWrite  DataStoreName=AcousticPose3
  Output Heirarchy : Subsystem
  Ping Point : MATLAB Function  TreatAsAtomicUnit=on
  Outputs : Outport
  Finished : Outport  Port=2
  wires:
  Sensors/1 -> Output Heirarchy/2(Sensors), Bus Selector/1
  Ping Point/3(Data) -> Output Heirarchy/1(Data)
  Output Heirarchy/1(Outputs) -> Outputs/1
  Bus Selector/3 -> Ping Point/3(Y)  "<Y>"
  Bus Selector/2 -> Ping Point/2(X)  "<X>"
  Bus Selector/4 -> Ping Point/4(Psi)  "<Psi>"
  Bus Selector/5 -> Ping Point/5(HorizBearing)  "<Horizontal Bearing>"
  Ping Point/2(Finished) -> Finished/1
  Ping Point/1(acousticPose) -> Data Store Write/1
  Bus Selector/1 -> Ping Point/1(Deployed)  "<Deployed>"
  Bus Selector/6 -> Ping Point/6(ElapsedTime)  "<Elapsed Time>"

== system RobotX_ss_acoustics_1019_bbox/Main FSM/Acoustic FSM/Move 1 ==
  Sensors : Inport
  Enable : EnablePort
  Bus Selector : BusSelector  OutputSignals=Navigation Message.Pose.X,Navigation Message.Pose.Y,Navigation Message.Pose.Psi,Navigation Message.Velocity.u
  CalcTimes : MATLAB Function  TreatAsAtomicUnit=on
  Data Store Read : DataStoreRead  DataStoreName=acouLocNED
  GPSMove : MATLAB Function  TreatAsAtomicUnit=on
  Output Reassign : Subsystem
  Submatrix : dspmtrx3/Submatrix  RowSpan=One row  RowStartMode=First  RowStartIndex=1  RowEndMode=Last  RowEndIndex=1  ColSpan=All columns  ColStartMode=First  ColStartIndex=1  ColEndMode=Last  ColEndIndex=1
  Outputs : Outport
  Finished : Outport  Port=2
  wires:
  GPSMove/3(pts) -> CalcTimes/1(pts)
  Sensors/1 -> Output Reassign/3(Sensors), Bus Selector/1
  Bus Selector/1 -> GPSMove/2(X)  "<X>"
  Bus Selector/2 -> GPSMove/3(Y)  "<Y>"
  Bus Selector/3 -> GPSMove/4(Psi)  "<Psi>"
  Bus Selector/4 -> CalcTimes/2(u)  "<u>"
  GPSMove/1(Finished) -> Finished/1
  Output Reassign/1(Outputs) -> Outputs/1
  CalcTimes/1(Data) -> Output Reassign/2(Data)
  GPSMove/2(valid) -> Output Reassign/1(Vaild)
  Submatrix/1 -> GPSMove/1(GoalNED)
  Data Store Read/1 -> Submatrix/1

== system RobotX_ss_acoustics_1019_bbox/Main FSM/Acoustic FSM/Move 2 ==
  Sensors : Inport
  Enable : EnablePort
  Bus Selector : BusSelector  OutputSignals=Navigation Message.Pose.X,Navigation Message.Pose.Y,Navigation Message.Pose.Psi,Navigation Message.Velocity.u
  CalcTimes : MATLAB Function  TreatAsAtomicUnit=on
  Data Store Read : DataStoreRead  DataStoreName=acouLocNED
  GPSMove : MATLAB Function  TreatAsAtomicUnit=on
  Output Reassign : Subsystem
  Submatrix : dspmtrx3/Submatrix  RowSpan=One row  RowStartMode=Middle  RowStartIndex=1  RowEndMode=Last  RowEndIndex=1  ColSpan=All columns  ColStartMode=First  ColStartIndex=1  ColEndMode=Last  ColEndIndex=1
  Outputs : Outport
  Finished : Outport  Port=2
  wires:
  GPSMove/3(pts) -> CalcTimes/1(pts)
  Sensors/1 -> Output Reassign/3(Sensors), Bus Selector/1
  Bus Selector/1 -> GPSMove/2(X)  "<X>"
  Bus Selector/2 -> GPSMove/3(Y)  "<Y>"
  Bus Selector/3 -> GPSMove/4(Psi)  "<Psi>"
  Bus Selector/4 -> CalcTimes/2(u)  "<u>"
  GPSMove/1(Finished) -> Finished/1
  Output Reassign/1(Outputs) -> Outputs/1
  CalcTimes/1(Data) -> Output Reassign/2(Data)
  GPSMove/2(valid) -> Output Reassign/1(Vaild)
  Submatrix/1 -> GPSMove/1(GoalNED)
  Data Store Read/1 -> Submatrix/1

== system RobotX_ss_acoustics_1019_bbox/Main FSM/Acoustic FSM/Move 3 ==
  Sensors : Inport
  Enable : EnablePort
  Bus Selector : BusSelector  OutputSignals=Navigation Message.Pose.X,Navigation Message.Pose.Y,Navigation Message.Pose.Psi,Navigation Message.Velocity.u
  CalcTimes : MATLAB Function  TreatAsAtomicUnit=on
  Data Store Read : DataStoreRead  DataStoreName=acouLocNED
  GPSMove : MATLAB Function  TreatAsAtomicUnit=on
  Output Reassign : Subsystem
  Submatrix : dspmtrx3/Submatrix  RowSpan=One row  RowStartMode=Last  RowStartIndex=1  RowEndMode=Last  RowEndIndex=1  ColSpan=All columns  ColStartMode=First  ColStartIndex=1  ColEndMode=Last  ColEndIndex=1
  Outputs : Outport
  Finished : Outport  Port=2
  wires:
  GPSMove/3(pts) -> CalcTimes/1(pts)
  Sensors/1 -> Output Reassign/3(Sensors), Bus Selector/1
  Bus Selector/1 -> GPSMove/2(X)  "<X>"
  Bus Selector/2 -> GPSMove/3(Y)  "<Y>"
  Bus Selector/3 -> GPSMove/4(Psi)  "<Psi>"
  Bus Selector/4 -> CalcTimes/2(u)  "<u>"
  GPSMove/1(Finished) -> Finished/1
  Output Reassign/1(Outputs) -> Outputs/1
  CalcTimes/1(Data) -> Output Reassign/2(Data)
  GPSMove/2(valid) -> Output Reassign/1(Vaild)
  Submatrix/1 -> GPSMove/1(GoalNED)
  Data Store Read/1 -> Submatrix/1

== system RobotX_ss_acoustics_1019_bbox/Main FSM/Acoustic FSM/Point ==
  Sensors : Inport
  Enable : EnablePort
  Bus Selector : BusSelector  OutputSignals=Navigation Message.Pose.X,Navigation Message.Pose.Y
  Data Store Read : DataStoreRead  DataStoreName=AcousticPose1
  Data Store Read1 : DataStoreRead  DataStoreName=AcousticPose2
  Data Store Read2 : DataStoreRead  DataStoreName=AcousticPose3
  Output Heirarchy : Subsystem
  Point : MATLAB Function  TreatAsAtomicUnit=on
  Outputs : Outport
  wires:
  Sensors/1 -> Output Heirarchy/2(Sensors), Bus Selector/1
  Point/1(Data) -> Output Heirarchy/1(Data)
  Output Heirarchy/1(Outputs) -> Outputs/1
  Bus Selector/1 -> Point/4(X)  "<X>"
  Bus Selector/2 -> Point/5(Y)  "<Y>"
  Data Store Read/1 -> Point/1(AcousticPose1)
  Data Store Read1/1 -> Point/2(AcousticPose2)
  Data Store Read2/1 -> Point/3(AcousticPose3)

== system RobotX_ss_acoustics_1019_bbox/Main FSM/Initialization/Output Heirarchy ==
  Sensors : Inport
  Acoustic Active : Constant  Value=0
  Bus Creator1 : BusCreator  Inputs=3
  Bus Creator2 : BusCreator  Inputs=3
  Bus Creator4 : BusCreator  Inputs=2
  Constant : Constant  Value=0
  Constant1 : Constant  Value=0
  Constant2 : Constant  Value=zeros(24,1)
  Lidar Mode : Constant  Value=0
  Outputs : Outport
  wires:
  Sensors/1 -> Bus Creator4/2  "Sensors"
  Bus Creator4/1 -> Outputs/1  "Output Signals"
  Constant/1 -> Bus Creator1/1  "Valid"
  Constant1/1 -> Bus Creator1/2  "Control Mode"
  Constant2/1 -> Bus Creator1/3  "Data"
  Bus Creator1/1 -> Bus Creator2/1  "Navigation Outputs"
  Acoustic Active/1 -> Bus Creator2/2  "Acoustic Active"
  Lidar Mode/1 -> Bus Creator2/3  "Lidar Mode"
  Bus Creator2/1 -> Bus Creator4/1  "Outputs"

== system RobotX_ss_acoustics_1019_bbox/Main FSM/RCHold/Direct Control ==
  Sensors : Inport
  Acoustic Active : Constant  Value=0
  Bus Creator2 : BusCreator  Inputs=3
  Bus Creator3 : BusCreator  Inputs=3
  Bus Creator4 : BusCreator  Inputs=2
  Constant : Constant
  Constant1 : Constant  Value=2
  Constant2 : Constant  Value=zeros(24,1)
  Lidar Mode : Constant  Value=3
  Outputs : Outport
  wires:
  Sensors/1 -> Bus Creator4/2  "Sensors"
  Bus Creator4/1 -> Outputs/1  "Output Signals"
  Bus Creator2/1 -> Bus Creator3/1  "Navigation Outputs"
  Acoustic Active/1 -> Bus Creator3/2  "Acoustic Active"
  Lidar Mode/1 -> Bus Creator3/3  "Lidar Mode"
  Bus Creator3/1 -> Bus Creator4/1  "Outputs"
  Constant/1 -> Bus Creator2/1  "Valid"
  Constant1/1 -> Bus Creator2/2  "Control Mode"
  Constant2/1 -> Bus Creator2/3  "Data"

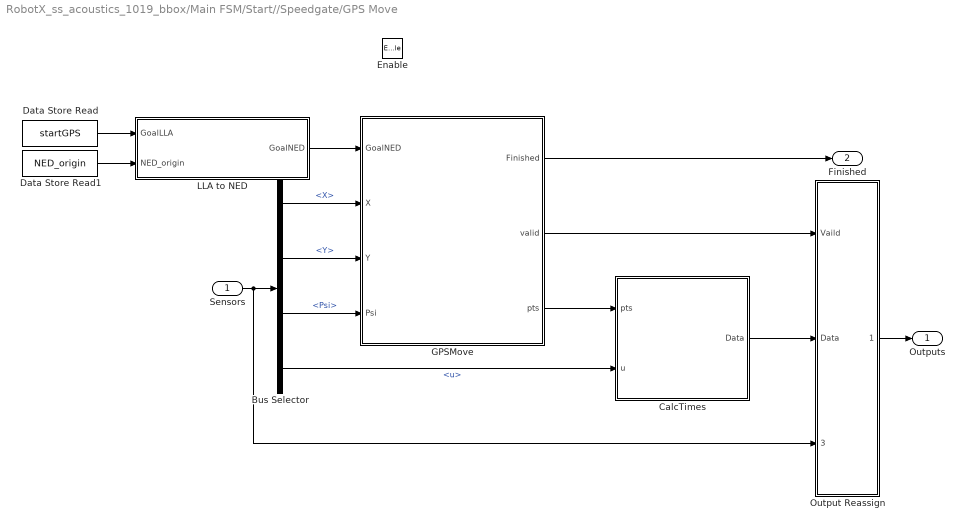
== system RobotX_ss_acoustics_1019_bbox/Main FSM/Start//Speedgate/GPS Move ==
  Sensors : Inport
  Enable : EnablePort
  Bus Selector : BusSelector  OutputSignals=Navigation Message.Pose.X,Navigation Message.Pose.Y,Navigation Message.Pose.Psi,Navigation Message.Velocity.u
  CalcTimes : MATLAB Function  TreatAsAtomicUnit=on
  Data Store Read : DataStoreRead  DataStoreName=startGPS
  Data Store Read1 : DataStoreRead  DataStoreName=NED_origin
  GPSMove : MATLAB Function  TreatAsAtomicUnit=on
  LLA to NED : MATLAB Function  TreatAsAtomicUnit=on
  Output Reassign : Subsystem
  Outputs : Outport
  Finished : Outport  Port=2
  wires:
  GPSMove/3(pts) -> CalcTimes/1(pts)
  Sensors/1 -> Output Reassign/3(Sensors), Bus Selector/1
  Bus Selector/1 -> GPSMove/2(X)  "<X>"
  Bus Selector/2 -> GPSMove/3(Y)  "<Y>"
  Bus Selector/3 -> GPSMove/4(Psi)  "<Psi>"
  Bus Selector/4 -> CalcTimes/2(u)  "<u>"
  GPSMove/1(Finished) -> Finished/1
  Output Reassign/1(Outputs) -> Outputs/1
  CalcTimes/1(Data) -> Output Reassign/2(Data)
  GPSMove/2(valid) -> Output Reassign/1(Vaild)
  LLA to NED/1(GoalNED) -> GPSMove/1(GoalNED)
  Data Store Read/1 -> LLA to NED/1(GoalLLA)
  Data Store Read1/1 -> LLA to NED/2(NED_origin)

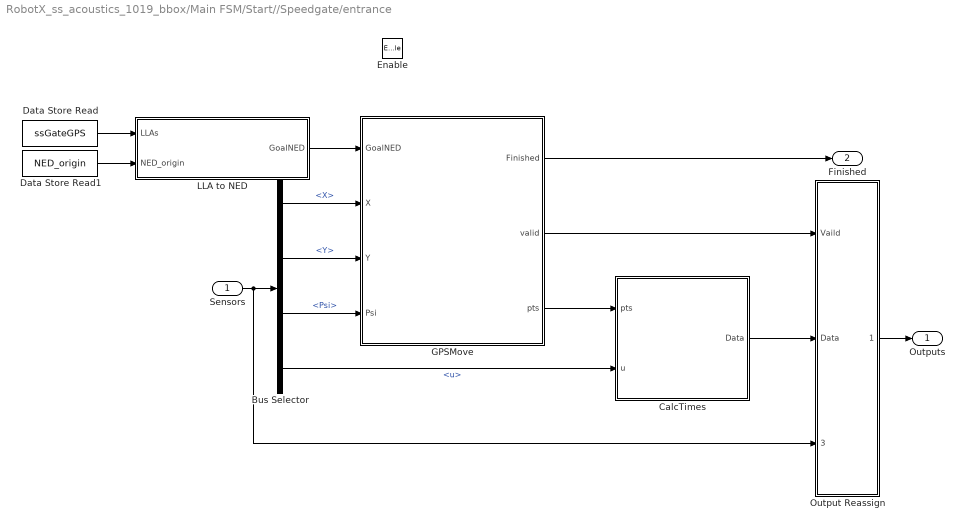
== system RobotX_ss_acoustics_1019_bbox/Main FSM/Start//Speedgate/entrance ==
  Sensors : Inport
  Enable : EnablePort
  Bus Selector : BusSelector  OutputSignals=Navigation Message.Pose.X,Navigation Message.Pose.Y,Navigation Message.Pose.Psi,Navigation Message.Velocity.u
  CalcTimes : MATLAB Function  TreatAsAtomicUnit=on
  Data Store Read : DataStoreRead  DataStoreName=ssGateGPS
  Data Store Read1 : DataStoreRead  DataStoreName=NED_origin
  GPSMove : MATLAB Function  TreatAsAtomicUnit=on
  LLA to NED : MATLAB Function  TreatAsAtomicUnit=on
  Output Reassign : Subsystem
  Outputs : Outport
  Finished : Outport  Port=2
  wires:
  GPSMove/3(pts) -> CalcTimes/1(pts)
  Sensors/1 -> Output Reassign/3(Sensors), Bus Selector/1
  Bus Selector/1 -> GPSMove/2(X)  "<X>"
  Bus Selector/2 -> GPSMove/3(Y)  "<Y>"
  Bus Selector/3 -> GPSMove/4(Psi)  "<Psi>"
  Bus Selector/4 -> CalcTimes/2(u)  "<u>"
  GPSMove/1(Finished) -> Finished/1
  Output Reassign/1(Outputs) -> Outputs/1
  CalcTimes/1(Data) -> Output Reassign/2(Data)
  GPSMove/2(valid) -> Output Reassign/1(Vaild)
  LLA to NED/1(GoalNED) -> GPSMove/1(GoalNED)
  Data Store Read/1 -> LLA to NED/1(LLAs)
  Data Store Read1/1 -> LLA to NED/2(NED_origin)

== system RobotX_ss_acoustics_1019_bbox/Main FSM/Start//Speedgate/exit ==
  Sensors : Inport
  Enable : EnablePort
  Bus Selector : BusSelector  OutputSignals=Navigation Message.Pose.X,Navigation Message.Pose.Y,Navigation Message.Pose.Psi,Navigation Message.Velocity.u
  CalcTimes : MATLAB Function  TreatAsAtomicUnit=on
  Data Store Read : DataStoreRead  DataStoreName=ssGateGPS
  Data Store Read1 : DataStoreRead  DataStoreName=NED_origin
  GPSMove : MATLAB Function  TreatAsAtomicUnit=on
  LLA to NED : MATLAB Function  TreatAsAtomicUnit=on
  Output Reassign : Subsystem
  Outputs : Outport
  Finished : Outport  Port=2
  wires:
  GPSMove/3(pts) -> CalcTimes/1(pts)
  Sensors/1 -> Output Reassign/3(Sensors), Bus Selector/1
  Bus Selector/1 -> GPSMove/2(X)  "<X>"
  Bus Selector/2 -> GPSMove/3(Y)  "<Y>"
  Bus Selector/3 -> GPSMove/4(Psi)  "<Psi>"
  Bus Selector/4 -> CalcTimes/2(u)  "<u>"
  GPSMove/1(Finished) -> Finished/1
  Output Reassign/1(Outputs) -> Outputs/1
  CalcTimes/1(Data) -> Output Reassign/2(Data)
  GPSMove/2(valid) -> Output Reassign/1(Vaild)
  LLA to NED/1(GoalNED) -> GPSMove/1(GoalNED)
  Data Store Read/1 -> LLA to NED/1(LLAs)
  Data Store Read1/1 -> LLA to NED/2(NED_origin)

== system RobotX_ss_acoustics_1019_bbox/Main FSM/Termination/Output Reassign ==
  Vaild : Inport
  Data : Inport  Port=2
  Sensors : Inport  Port=3
  Acoustic Active : Constant  Value=0
  Bus Creator2 : BusCreator  Inputs=3
  Bus Creator3 : BusCreator  Inputs=3
  Bus Creator5 : BusCreator  Inputs=2
  Constant3 : Constant  Value=0
  Lidar Mode : Constant  Value=0
  Outputs : Outport
  wires:
  Sensors/1 -> Bus Creator5/2  "Sensors"
  Bus Creator5/1 -> Outputs/1  "Output Signals"
  Vaild/1 -> Bus Creator2/1  "Valid"
  Constant3/1 -> Bus Creator2/2  "Control Mode"
  Data/1 -> Bus Creator2/3  "Data"
  Bus Creator2/1 -> Bus Creator3/1  "Navigation Outputs"
  Acoustic Active/1 -> Bus Creator3/2  "Acoustic Active"
  Lidar Mode/1 -> Bus Creator3/3  "Lidar Mode"
  Bus Creator3/1 -> Bus Creator5/1  "Outputs"

== system RobotX_ss_acoustics_1019_bbox/Sensors/Serial In/ Raspberry Pi LCM (Acoustic) ==
  LCM Input : Inport
  ASCII Decode 6 : xpcseriallib/ASCII Decode   format=Deploy:%1u, Elapsed:%g, Bearing1:%g Bearing2:%g \r\n  nvars=4  vartypes={}
  Bus Creator : BusCreator  Inputs=2
  Bus Creator1 : BusCreator  Inputs=3
  FIFO ASCII read 1 : xpcseriallib/FIFO ASCII read   header={'Deploy:'}  term=[13 10]  hold=Zero output if no new data  enable=off  maxsize=1024  outputtype=8 bit uint null terminated  sampletime=-1
  LCM Output : Outport
  wires:
  LCM Input/1 -> FIFO ASCII read 1/1
  FIFO ASCII read 1/1 -> ASCII Decode 6/1
  ASCII Decode 6/3 -> Bus Creator/1  "Horizontal Bearing"
  ASCII Decode 6/4 -> Bus Creator/2  "Vertical Bearing"
  Bus Creator/1 -> Bus Creator1/3  "Bearings"
  ASCII Decode 6/2 -> Bus Creator1/2  "Elapsed Time"
  ASCII Decode 6/1 -> Bus Creator1/1  "Deployed"
  Bus Creator1/1 -> LCM Output/1  "Acoustic Message"

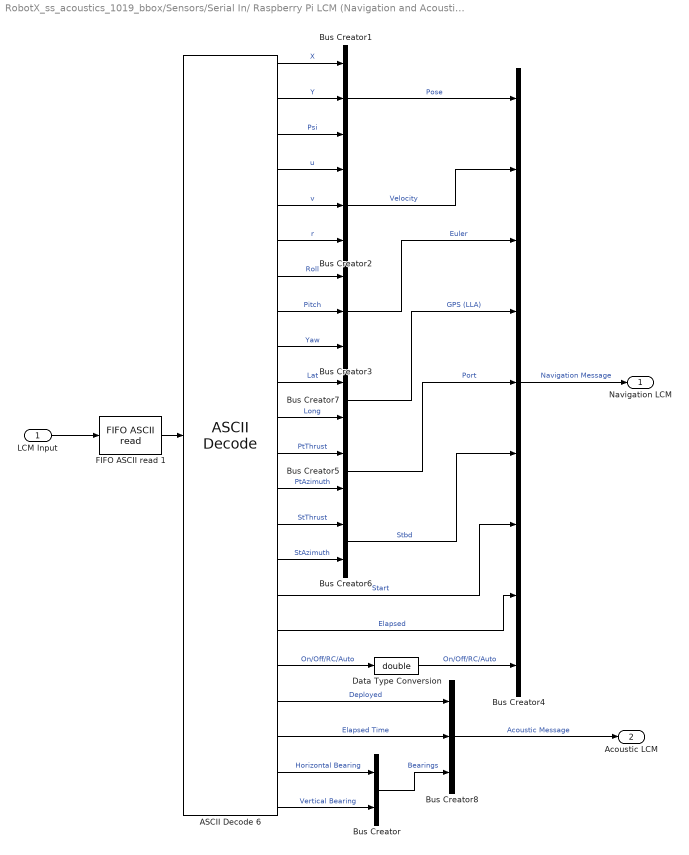
== system RobotX_ss_acoustics_1019_bbox/Sensors/Serial In/ Raspberry Pi LCM (Navigation and Acoustics) ==
  LCM Input : Inport
  ASCII Decode 6 : xpcseriallib/ASCII Decode   format=P1:%f P2:%f P3:%f V1:%f V2:%f V3:%f E1:%f E2:%f E3:%f Pt1:%f Pt2:%f St1:%f St2:%f Start:%f Elapsed:%f RC:%d Deploy:%u, Elapsed:%g, Bearing1:%g Bearing2:%g \r\n  nvars=22  vartypes={}
  Bus Creator{,5..7} (4 alike) : BusCreator  Inputs=2
  Bus Creator{1..3,8} (4 alike) : BusCreator  Inputs=3
  Bus Creator4 : BusCreator  Inputs=9
  Data Type Conversion : DataTypeConversion  OutDataTypeStr=double
  FIFO ASCII read 1 : xpcseriallib/FIFO ASCII read   header={'P1:'}  term=[13 10]  hold=Zero output if no new data  enable=off  maxsize=2048  outputtype=8 bit uint null terminated  sampletime=-1
  Navigation LCM : Outport
  Acoustic LCM : Outport  Port=2
  wires:
  LCM Input/1 -> FIFO ASCII read 1/1
  FIFO ASCII read 1/1 -> ASCII Decode 6/1
  Bus Creator4/1 -> Navigation LCM/1  "Navigation Message"
  ASCII Decode 6/1 -> Bus Creator1/1  "X"
  ASCII Decode 6/2 -> Bus Creator1/2  "Y"
  ASCII Decode 6/3 -> Bus Creator1/3  "Psi"
  Bus Creator1/1 -> Bus Creator4/1  "Pose"
  ASCII Decode 6/4 -> Bus Creator2/1  "u"
  ASCII Decode 6/5 -> Bus Creator2/2  "v"
  Bus Creator2/1 -> Bus Creator4/2  "Velocity"
  ASCII Decode 6/7 -> Bus Creator3/1  "Roll"
  ASCII Decode 6/8 -> Bus Creator3/2  "Pitch"
  ASCII Decode 6/9 -> Bus Creator3/3  "Yaw"
  Bus Creator3/1 -> Bus Creator4/3  "Euler"
  Bus Creator5/1 -> Bus Creator4/5  "Port"
  Bus Creator6/1 -> Bus Creator4/6  "Stbd"
  ASCII Decode 6/14 -> Bus Creator6/1  "StThrust"
  ASCII Decode 6/15 -> Bus Creator6/2  "StAzimuth"
  ASCII Decode 6/12 -> Bus Creator5/1  "PtThrust"
  ASCII Decode 6/13 -> Bus Creator5/2  "PtAzimuth"
  ASCII Decode 6/16 -> Bus Creator4/7  "Start"
  ASCII Decode 6/17 -> Bus Creator4/8  "Elapsed"
  ASCII Decode 6/18 -> Data Type Conversion/1  "On/Off/RC/Auto"
  Data Type Conversion/1 -> Bus Creator4/9  "On/Off/RC/Auto"
  ASCII Decode 6/6 -> Bus Creator2/3  "r"
  ASCII Decode 6/10 -> Bus Creator7/1  "Lat"
  ASCII Decode 6/11 -> Bus Creator7/2  "Long"
  Bus Creator7/1 -> Bus Creator4/4  "GPS (LLA)"
  ASCII Decode 6/21 -> Bus Creator/1  "Horizontal Bearing"
  ASCII Decode 6/22 -> Bus Creator/2  "Vertical Bearing"
  Bus Creator/1 -> Bus Creator8/3  "Bearings"
  ASCII Decode 6/20 -> Bus Creator8/2  "Elapsed Time"
  ASCII Decode 6/19 -> Bus Creator8/1  "Deployed"
  Bus Creator8/1 -> Acoustic LCM/1  "Acoustic Message"
